simulink model "Circuit_3State_Overall"  (R2022a)
settings: Solver=VariableStepAuto  StartTime=0.0  StopTime=10.0  RelTol=1e-3
model workspace (MAT data in the model file):
  A = [-1  0.5  0; -0.5  1  -0.5; 0  0.5  -1]
  A_ROM = [0.00190368543086  0.0382121709593; 0.0255020998729  0.511896862984]
  B = [0.5; 0; 0]
  B_ROM = [6.0644019285; 7.56779179745]
  C_des = [1  0  0; 0  1  0; 0  0  1]
  C_des_ROM = [0.121212121212  -0.00378787878788; 0.0607908351811  0.00591278640059; 0.000369549150037  0.0156134515891]
  C_m = [0 0 1]
  C_m_ROM = [0.000369549150037 0.0156134515891]
  FLAG.Analysis.NoNoiseCompare = 0
  FLAG.Analysis.ode3 = 1
  FLAG.Analysis.ode5 = 1
  FLAG.Analysis.SS_CT3 = 1
  FLAG.Analysis.SS_DT3 = 1
  FLAG.Analysis.ROM_Mlab3 = 1
  FLAG.Analysis.ROM_HoKal = 0
  FLAG.Analysis.NoisyPlant = 1
  FLAG.Analysis.Estimator = 1
  FLAG.Analysis.Est_Error_calc = 1
  FLAG.Analysis.GenComparData = 1
  FLAG.Analysis.ComparSVD2Pinf = 0
  FLAG.PLOT.PlotResults = 0
  FLAG.C_mode = 3
  FLAG.QMode = 1
  FLAG.InputMode = 1
  FLAG.SlinkModel = 3
  FLAG.EstimatorModel = 1
  FLAG.InputSignalMode = 2
  InputSignal = [0  4; 0.0001  4; 0.0002  4; 0.0003  4]
  K_plant = [0  0  0; 0  10000000  0; 0  0  0]
  M_cross = [1000000  0  0; 0  0  0; 0  0  10000]
  N.measur = 1
  N.inputs = 1
  N.states = 3
  P.V_1 = 1
  P.V_2 = 2
  P.V_3 = 3
  P.V_s = 4
  P.i_PS = 5
  SIM.AnalysisComplete.Initialization = 0
  SIM.AnalysisComplete.NoNoiseCompare.ode3 = 0
  SIM.AnalysisComplete.NoNoiseCompare.ode5 = 0
  SIM.AnalysisComplete.NoNoiseCompare.SS_CT3 = 0
  SIM.AnalysisComplete.NoNoiseCompare.SS_DT3 = 0
  SIM.AnalysisComplete.NoNoiseCompare.ROM_Mlab3 = 0
  SIM.AnalysisComplete.NoNoiseCompare.ROM_HoKal = 0
  SIM.AnalysisComplete.NoisyPlant = 0
  SIM.AnalysisComplete.Estimator = 0
  SIM.AnalysisComplete.Est_Error_calc = 0
  SIM.AnalysisComplete.GenComparData = 0
  SIM.AnalysisComplete.ComparSVD2Pinf = 0
  SIM.Analysis.OverwriteData = 1
  SIM.Analysis.NoisyPlant.OverwriteData = 1
  SIM.Ts = 0.0001
  SIM.tc = 0.0001
  SIM.Q_0 = 10
  SIM.R_0 = 10
  SIM.V_init = 0
  SIM.V_step_height = 4
  SIM.fq = 400
  SIM.V_s = 1
  SIM.t_final = 0.0001
  SIM.save_filename = 'F:\TylerFiles\GitHubRepos\BatteryModel\Model\KalmanTesting\DAE_Circuit\SoftwareStyle\Results\Plant_Step_InputQ_Q10_R10_Ts0.0001_C3.mat'
  SIM.C_1 = 1e-06
  SIM.C_4 = 0.0001
  SIM.R_1 = 2
  SIM.R_2 = 2
  SIM.R_3 = 2
  SIM.R_4 = 2
  SIM.Mass3 = [1e-06  0  0; 0  0  0; 0  0  0.0001]
  SIM.algb_idx3 = 2
  SIM.diff_idx3 = [1 3]
  SIM.Mass5 = [1e-06  0  0  -1e-06  0; 0  0  0  0  0; 0  0  0.0001  0  0; -1e-06  0  0  1e-06  0; 0  0  0  0  0]
  SIM.algb_idx5 = [2 5]
  SIM.diff_idx5 = [1 3 4]
  SIM.V_step = 4
  SIM.time_rest = 0
  SIM.time_ramp = 2e-05
  SIM.t_final_sim = 0.0003
  SIM.t_vec = [0 0.0001 0.0002 0.0003]
  SIM.omega = 2513.27412287
  SIM.x_0_3 = [4; 2; 0]
  SIM.x_0_5 = [0; 0; 0; 0; 0]
  SIM.Q3i = 10
  SIM.Q5i = 10
  SIM.Q3s = [10; 10; 10]
  SIM.Q5s = [10 10 10 10 10]
  SIM.R = 10
  SIM.pow_Q3i = 0.001
  SIM.pow_Q5i = 0.001
  SIM.pow_Q3s = [0.001; 0.001; 0.001]
  SIM.pow_Q5s = [0.001 0.001 0.001 0.001 0.001]
  SIM.pow_R = 0.001
  SV_IC = [4; 2; 0]
  Ts = 0.0001
  U_NV_NT = [0  0  0; 0  1  0; 0  0  0]
  pow_Q3i = 0.001
  pow_R = 0.001
  tc = 0.0001
  x_0_ROM = [32.9756097561; -0.780487804878]
settings Model: Creator=tyevans  LastModifiedBy=tyevans

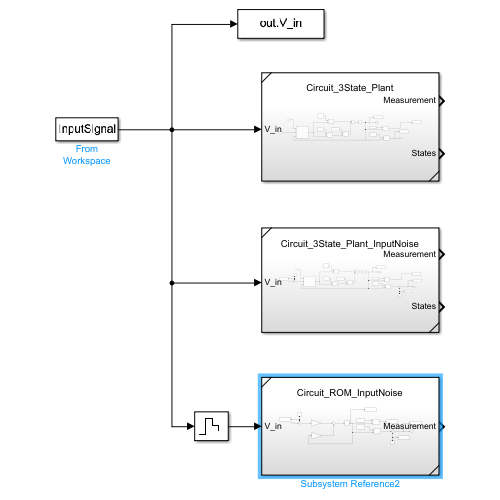
[thumbnail: Simulink's stored preview of the top-level diagram]
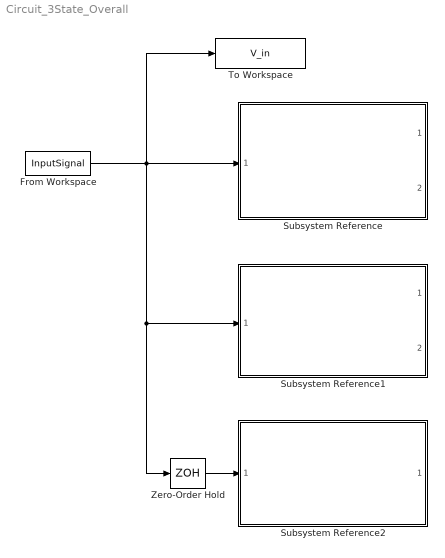
== system Circuit_3State_Overall ==
  From Workspace : FromWorkspace  VariableName=InputSignal  OutputAfterFinalValue=Setting to zero
  Subsystem Reference : Subsystem  ReferencedSubsystem=Circuit_3State_Plant
  Subsystem Reference1 : Subsystem  ReferencedSubsystem=Circuit_3State_Plant_InputNoise
  Subsystem Reference2 : Subsystem  ReferencedSubsystem=Circuit_ROM_InputNoise
  To Workspace : ToWorkspace  VariableName=V_in  SaveFormat=Structure With Time  SampleTime=Ts
  Zero-Order Hold : ZeroOrderHold  SampleTime=Ts
  wires:
  From Workspace/1 -> Subsystem Reference/1, To Workspace/1, Subsystem Reference1/1, Zero-Order Hold/1
  Zero-Order Hold/1 -> Subsystem Reference2/1
